simulink model "Lab_1_Simulation_Model_2021a"  (R2021a)
settings: Solver=VariableStepAuto  StartTime=0.0  StopTime=20  RelTol=1e-3
values from neighbouring files (symbols this model uses):
  Constant_Disturbance = 0    [Lab_1_Simulation_TA(1).m]    (also in Lab_1_Simulation_TA.m)
  Disturbance_Frequency = 1    [Lab_1_Simulation_TA(1).m]    (also in Lab_1_Simulation_TA.m)
  Sine_Disturbance = 0    [Lab_1_Simulation_TA(1).m]    (also in Lab_1_Simulation_TA.m)
  Square_Frequency = 1    [Lab_1_Simulation_TA(1).m]    (also in Lab_1_Simulation_TA.m)
  Square_Size = 0    [Lab_1_Simulation_TA(1).m]    (also in Lab_1_Simulation_TA.m)
  Step_Size = 40    [Lab_1_Simulation_TA(1).m]    (also in Lab_1_Simulation_TA.m)
  Step_Time = 0    [Lab_1_Simulation_TA(1).m]    (also in Lab_1_Simulation_TA.m = 10)
libraries: cstblocks x2
settings Model: Creator=20193255  LastModifiedBy=20193255
settings DebuggingCC: UnconnectedInputMsg=none  UnconnectedOutputMsg=none  UnconnectedLineMsg=none
settings ModelReferenceCC: EnableRefExpFcnMdlSchedulingChecks=off
settings RTWCC: Description=Generic Real-Time Target  GPUComputeCapability=5.0  DLArmComputeVersion=20.02.1

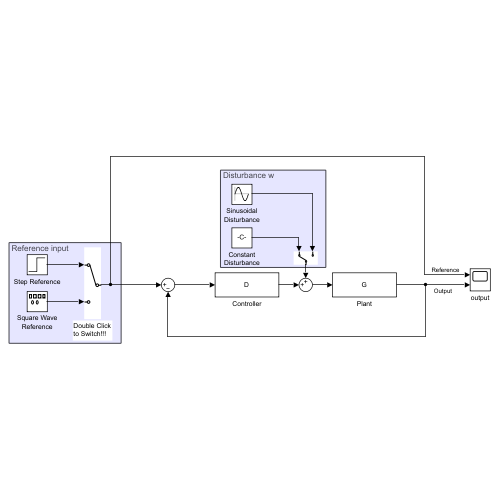
[thumbnail: Simulink's stored preview of the top-level diagram]
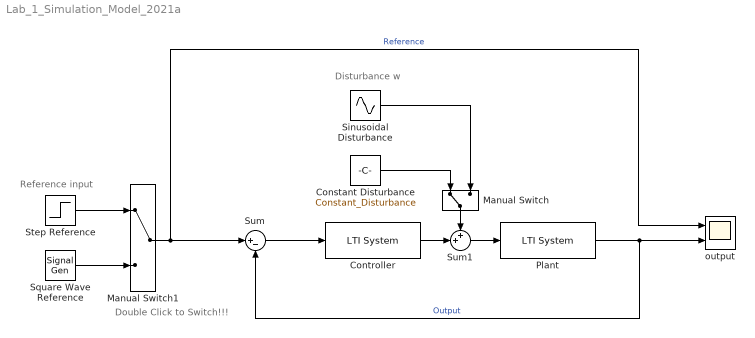
== system Lab_1_Simulation_Model_2021a ==
  note: Double Click to Switch!!!
  note: Disturbance w
  note: Reference input
  Constant Disturbance : Constant  Value=Constant_Disturbance
  Controller : cstblocks/LTI System  sys=D  IC=[]
  Manual Switch : ManualSwitch
  Manual Switch1 : ManualSwitch
  Plant : cstblocks/LTI System  sys=G  IC=[]
  Sinusoidal Disturbance : Sin  Amplitude=Sine_Disturbance  Frequency=Disturbance_Frequency  SampleTime=0
  Square Wave Reference : SignalGenerator  WaveForm=square  Amplitude=Square_Size  Frequency=Square_Frequency  Units=rad/sec
  Step Reference : Step  Time=Step_Time  After=Step_Size  SampleTime=0
  Sum : Sum  Inputs=|+-
  Sum1 : Sum  Inputs=++|
  output : Scope  NumInputPorts=2
  wires:
  Sum/1 -> Controller/1
  Plant/1 -> Sum/2, output/2  "Output"
  Manual Switch1/1 -> Sum/1, output/1  "Reference"
  Controller/1 -> Sum1/2
  Sum1/1 -> Plant/1
  Sinusoidal Disturbance/1 -> Manual Switch/2
  Constant Disturbance/1 -> Manual Switch/1
  Manual Switch/1 -> Sum1/1
  Step Reference/1 -> Manual Switch1/1
  Square Wave Reference/1 -> Manual Switch1/2
